simulink model "lab9sim"  (R2020a)
settings: Solver=VariableStepAuto  StartTime=0.0  StopTime=80  RelTol=1e-3
libraries: simulink x1
settings Model: Creator=ariana  LastModifiedBy=ariana

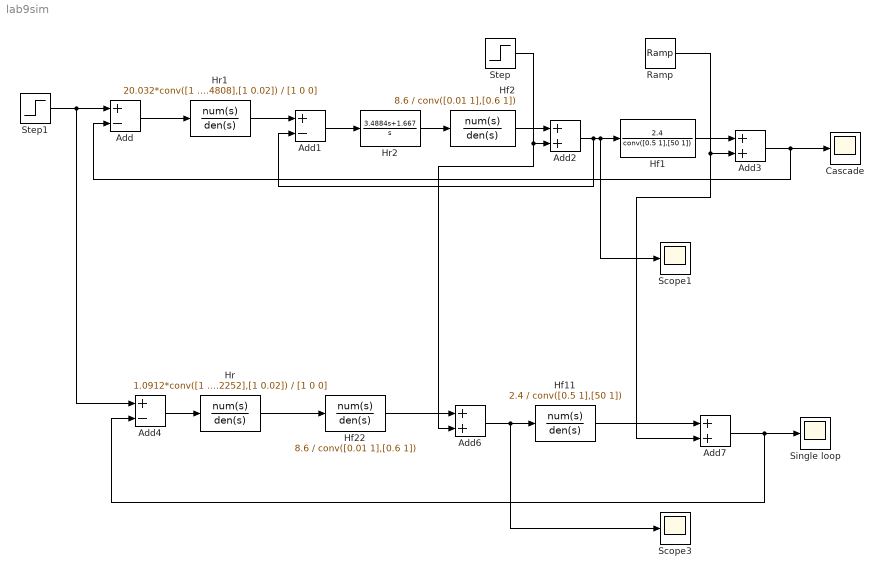
== system lab9sim ==
  " Hr" : TransferFcn  Numerator=1.0912*conv([1 0.2252],[1 0.02])  Denominator=[1 0 0]
  " Hr1" : TransferFcn  Numerator=20.032*conv([1 0.4808],[1 0.02])  Denominator=[1 0 0]
  " Hr2" : TransferFcn  Numerator=[3.4884 1.667]  Denominator=[1 0]
  Add : Sum  Inputs=+-
  Add1 : Sum  Inputs=+-
  Add{2..3,6..7} (4 alike) : Sum
  Add4 : Sum  Inputs=+-
  Cascade : Scope
  Hf1 : TransferFcn  Numerator=2.4  Denominator=conv([0.5 1],[50 1])
  Hf11 : TransferFcn  Numerator=2.4  Denominator=conv([0.5 1],[50 1])
  Hf2 : TransferFcn  Numerator=8.6  Denominator=conv([0.01 1],[0.6 1])
  Hf22 : TransferFcn  Numerator=8.6  Denominator=conv([0.01 1],[0.6 1])
  Ramp : simulink/Sources/Ramp  slope=1  start=50  InitialOutput=0
  Scope1 : Scope
  Scope3 : Scope
  Single loop : Scope
  Step : Step  Time=20  SampleTime=0
  Step1 : Step  Time=0  SampleTime=0
  wires:
  Add/1 -> " Hr1"/1
  " Hr1"/1 -> Add1/1
  Add1/1 -> " Hr2"/1
  " Hr2"/1 -> Hf2/1
  Add2/1 -> Add1/2, Scope1/1, Hf1/1
  Hf1/1 -> Add3/1
  Add3/1 -> Add/2, Cascade/1
  Hf2/1 -> Add2/1
  Hf22/1 -> Add6/1
  Add7/1 -> Add4/2, Single loop/1
  " Hr"/1 -> Hf22/1
  Step1/1 -> Add4/1, Add/1
  Add4/1 -> " Hr"/1
  Step/1 -> Add6/2, Add2/2
  Add6/1 -> Scope3/1, Hf11/1
  Hf11/1 -> Add7/1
  Ramp/1 -> Add7/2, Add3/2
